simulink model "Sim_braco"  (R2020a)
settings: Solver=VariableStepAuto  StartTime=0.0  StopTime=10.0  RelTol=1e-3
undefined symbols (not defined in the file or in its folder): H_b, H_c, H_o, pos_base, pos_coto, pos_ombro
settings Model: Creator=João Lula  LastModifiedBy=João Lula

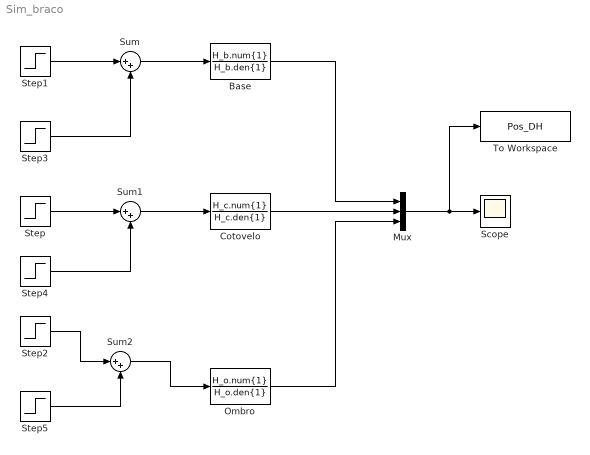
== system Sim_braco ==
  Base : TransferFcn  Numerator=H_b.num{1}  Denominator=H_b.den{1}
  Cotovelo : TransferFcn  Numerator=H_c.num{1}  Denominator=H_c.den{1}
  Mux : Mux  Inputs=3
  Ombro : TransferFcn  Numerator=H_o.num{1}  Denominator=H_o.den{1}
  Scope : Scope
  Step : Step  Time=5  After=pos_coto - 150  SampleTime=0
  Step1 : Step  Time=0  After=pos_base  SampleTime=0
  Step2 : Step  Time=5  After=pos_ombro - 150  SampleTime=0
  Step3 : Step  After=0  SampleTime=0
  Step4 : Step  Time=0  After=150  SampleTime=0
  Step5 : Step  Time=0  After=150  SampleTime=0
  Sum : Sum  Inputs=|++
  Sum1 : Sum  Inputs=|++
  Sum2 : Sum  Inputs=|++
  To Workspace : ToWorkspace  VariableName=Pos_DH  SaveFormat=Timeseries  SampleTime=-1
  wires:
  Base/1 -> Mux/1
  Cotovelo/1 -> Mux/2
  Ombro/1 -> Mux/3
  Mux/1 -> To Workspace/1, Scope/1
  Step1/1 -> Sum/1
  Sum/1 -> Base/1
  Step3/1 -> Sum/2
  Step/1 -> Sum1/1
  Sum1/1 -> Cotovelo/1
  Step4/1 -> Sum1/2
  Step2/1 -> Sum2/1
  Sum2/1 -> Ombro/1
  Step5/1 -> Sum2/2
